simulink model "asg1_3k03"  (R2019a)
settings: Solver=FixedStepAuto  StartTime=0.0  StopTime=100  FixedStep=1e-3  RelTol=1e-3  EnableMultiTasking=on
undefined symbols (not defined in the file): D0, D1, D10, D11, D12, D13, D2, D3, D4, D5, D6, D7, D8, D9, PTA0, PTA1, PTA2, PTB23, PTB9, PTC16, PTC17, PTC2, PTC3, PTC4, PTD0, PTD1, PTD2, PTD3, sigbuilder_block
libraries: frdmk64flib x20
settings Model: SimulationMode=external  ExtModeTrigDuration=5  Creator=Jinge Li  LastModifiedBy=Junbo Huang
settings DataIOCC: ReturnWorkspaceOutputs=off
settings OptimizationCC: EnhancedBackFolding=on  PassReuseOutputArgsAs=Individual arguments  MaxStackSize=64  OptimizeBlockOrder=speed  DifferentSizesBufferReuse=on  OptimizationCustomize=off
settings DebuggingCC: ParameterTunabilityLossMsg=error  ArithmeticOperatorsInVariantConditions=warning
settings HardwareCC: ProdBitPerPointer=32  ProdBitPerSizeT=32  ProdBitPerPtrDiffT=32  ProdLargestAtomicInteger=Long  ProdLargestAtomicFloat=Double  ProdWordSize=32  ProdHWDeviceType=ARM Compatible->ARM Cortex
settings SFSimCC: MATLABDynamicMemAlloc=off
settings RTWCC: SystemTargetFile=ert.tlc  HardwareBoard=NXP FRDM-K64F  TLCOptions="-aInlineSetEventsForThisBaseRateFcn=TLC_FALSE -aSuppressMultiTaskScheduler=TLC_FALSE  -aRateBasedStepFcn=0"  TemplateMakefile=ert_default_tmf  GenerateReport=on  Toolchain=GNU Tools for ARM Embedded Processors  IncludeHyperlinkInReport=on  LaunchReport=on  GenerateTraceInfo=on  GenerateTraceReport=on  GenerateTraceReportSl=on  GenerateTraceReportSf=on  GenerateTraceReportEml=on
settings CodeAppCC: ForceParamTrailComments=on  IgnoreCustomStorageClasses=off  OperatorAnnotations=on  SimulinkDataObjDesc=on  SFDataObjDesc=on  InsertBlockDesc=on
settings ERTTargetCC: SupportContinuousTime=on  ExtMode=on  ExtModeTransport=4  ExtModeMexFile=sendToCommService  ExtModeMexArgs='asg1_3k03' 0

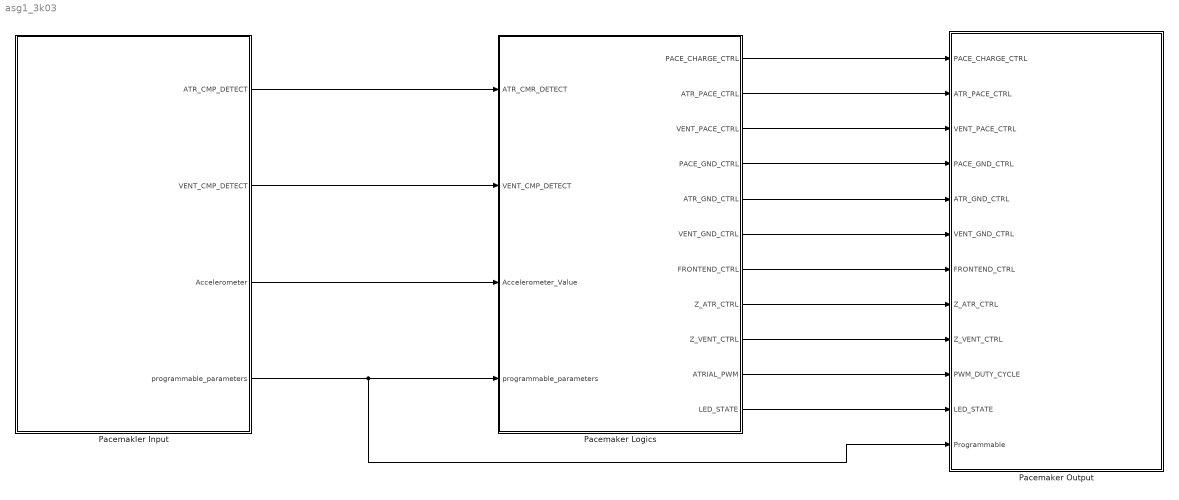
== system asg1_3k03 ==
  Pacemaker Logics : Subsystem
  Pacemaker Output : Subsystem
  Pacemakler Input : Subsystem
  wires:
  Pacemaker Logics/1(PACE_CHARGE_CTRL) -> Pacemaker Output/1(PACE_CHARGE_CTRL)
  Pacemaker Logics/3(VENT_PACE_CTRL) -> Pacemaker Output/3(VENT_PACE_CTRL)
  Pacemaker Logics/4(PACE_GND_CTRL) -> Pacemaker Output/4(PACE_GND_CTRL)
  Pacemaker Logics/5(ATR_GND_CTRL) -> Pacemaker Output/5(ATR_GND_CTRL)
  Pacemaker Logics/6(VENT_GND_CTRL) -> Pacemaker Output/6(VENT_GND_CTRL)
  Pacemakler Input/1(ATR_CMP_DETECT) -> Pacemaker Logics/1(ATR_CMR_DETECT)
  Pacemakler Input/2(VENT_CMP_DETECT) -> Pacemaker Logics/2(VENT_CMP_DETECT)
  Pacemaker Logics/2(ATR_PACE_CTRL) -> Pacemaker Output/2(ATR_PACE_CTRL)
  Pacemaker Logics/7(FRONTEND_CTRL) -> Pacemaker Output/7(FRONTEND_CTRL)
  Pacemakler Input/4(programmable_parameters) -> Pacemaker Output/12("Programmable "), Pacemaker Logics/4(programmable_parameters)
  Pacemaker Logics/8(Z_ATR_CTRL) -> Pacemaker Output/8(Z_ATR_CTRL)
  Pacemaker Logics/9(Z_VENT_CTRL) -> Pacemaker Output/9(Z_VENT_CTRL)
  Pacemaker Logics/10(ATRIAL_PWM) -> Pacemaker Output/10(PWM_DUTY_CYCLE)
  Pacemakler Input/3("Accelerometer ") -> Pacemaker Logics/3(Accelerometer_Value)
  Pacemaker Logics/11(LED_STATE) -> Pacemaker Output/11(LED_STATE)

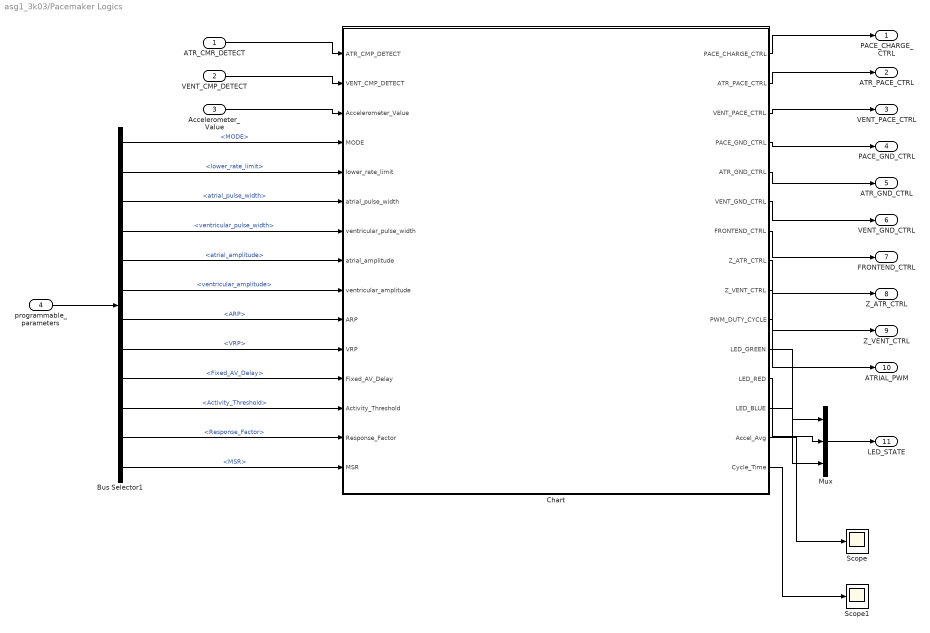
== system asg1_3k03/Pacemaker Logics ==
  ATR_CMR_DETECT : Inport
  VENT_CMP_DETECT : Inport  Port=2
  Accelerometer_Value : Inport  Port=3
  programmable_parameters : Inport  Port=4
  Bus Selector1 : BusSelector  OutputSignals=MODE,lower_rate_limit,atrial_pulse_width,ventricular_pulse_width,atrial_amplitude,ventricular_amplitude,ARP,VRP,Fixed_AV_Delay,Activity_Threshold,Response_Factor,MSR
  Chart : Stateflow chart  TreatAsAtomicUnit=on
  Mux : Mux  Inputs=3
  Scope : Scope
  Scope1 : Scope
  PACE_CHARGE_CTRL : Outport
  ATR_PACE_CTRL : Outport  Port=2
  VENT_PACE_CTRL : Outport  Port=3
  PACE_GND_CTRL : Outport  Port=4
  ATR_GND_CTRL : Outport  Port=5
  VENT_GND_CTRL : Outport  Port=6
  FRONTEND_CTRL : Outport  Port=7
  Z_ATR_CTRL : Outport  Port=8
  Z_VENT_CTRL : Outport  Port=9
  ATRIAL_PWM : Outport  Port=10
  LED_STATE : Outport  Port=11
  wires:
  Chart/1(PACE_CHARGE_CTRL) -> PACE_CHARGE_CTRL/1
  Bus Selector1/7 -> Chart/10(ARP)  "<ARP>"
  Bus Selector1/8 -> Chart/11(VRP)  "<VRP>"
  Bus Selector1/4 -> Chart/7(ventricular_pulse_width)  "<ventricular_pulse_width>"
  Chart/2(ATR_PACE_CTRL) -> ATR_PACE_CTRL/1
  Bus Selector1/6 -> Chart/9(ventricular_amplitude)  "<ventricular_amplitude>"
  Bus Selector1/5 -> Chart/8(atrial_amplitude)  "<atrial_amplitude>"
  Bus Selector1/2 -> Chart/5(lower_rate_limit)  "<lower_rate_limit>"
  Chart/9(Z_VENT_CTRL) -> Z_VENT_CTRL/1
  Chart/8(Z_ATR_CTRL) -> Z_ATR_CTRL/1
  Chart/7(FRONTEND_CTRL) -> FRONTEND_CTRL/1
  programmable_parameters/1 -> Bus Selector1/1
  Bus Selector1/1 -> Chart/4(MODE)  "<MODE>"
  Bus Selector1/3 -> Chart/6(atrial_pulse_width)  "<atrial_pulse_width>"
  VENT_CMP_DETECT/1 -> Chart/2(VENT_CMP_DETECT)
  Chart/4(PACE_GND_CTRL) -> PACE_GND_CTRL/1
  Chart/5(ATR_GND_CTRL) -> ATR_GND_CTRL/1
  Chart/6(VENT_GND_CTRL) -> VENT_GND_CTRL/1
  ATR_CMR_DETECT/1 -> Chart/1(ATR_CMP_DETECT)
  Chart/3(VENT_PACE_CTRL) -> VENT_PACE_CTRL/1
  Chart/10(PWM_DUTY_CYCLE) -> ATRIAL_PWM/1
  Bus Selector1/9 -> Chart/12(Fixed_AV_Delay)  "<Fixed_AV_Delay>"
  Accelerometer_Value/1 -> Chart/3(Accelerometer_Value)
  Chart/11(LED_GREEN) -> Mux/1
  Chart/12(LED_RED) -> Mux/2
  Chart/13(LED_BLUE) -> Mux/3
  Mux/1 -> LED_STATE/1
  Bus Selector1/10 -> Chart/13(Activity_Threshold)  "<Activity_Threshold>"
  Bus Selector1/11 -> Chart/14(Response_Factor)  "<Response_Factor>"
  Chart/14(Accel_Avg) -> Scope/1
  Bus Selector1/12 -> Chart/15(MSR)  "<MSR>"
  Chart/15(Cycle_Time) -> Scope1/1

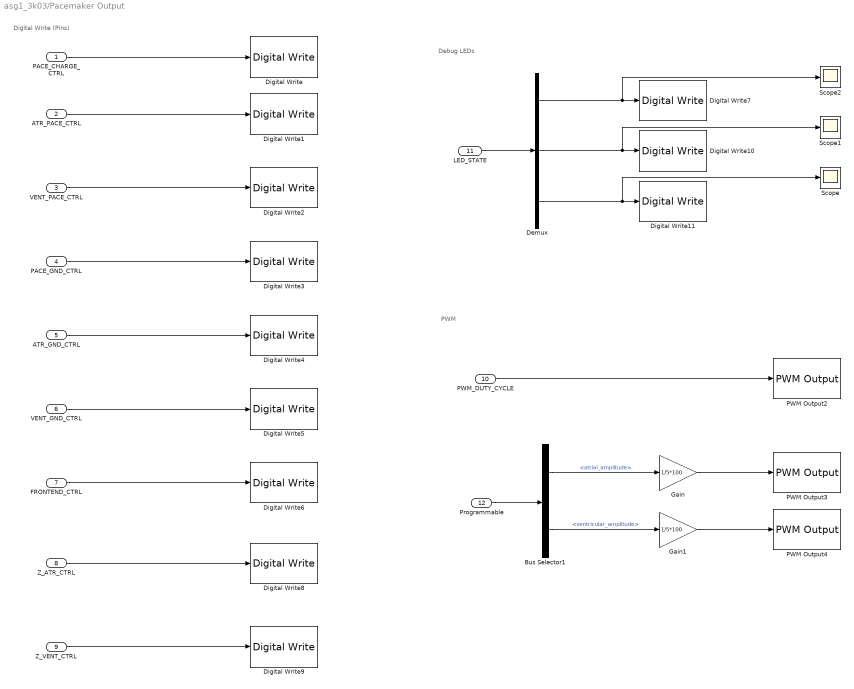
== system asg1_3k03/Pacemaker Output ==
  note: Digital Write (Pins)
  note: PWM
  note: Debug LEDs
  PACE_CHARGE_CTRL : Inport
  ATR_PACE_CTRL : Inport  Port=2
  VENT_PACE_CTRL : Inport  Port=3
  PACE_GND_CTRL : Inport  Port=4
  ATR_GND_CTRL : Inport  Port=5
  VENT_GND_CTRL : Inport  Port=6
  FRONTEND_CTRL : Inport  Port=7
  Z_ATR_CTRL : Inport  Port=8
  Z_VENT_CTRL : Inport  Port=9
  PWM_DUTY_CYCLE : Inport  Port=10
  LED_STATE : Inport  Port=11
  "Programmable " : Inport  Port=12
  Bus Selector1 : BusSelector  OutputSignals=atrial_amplitude,ventricular_amplitude
  Demux : Demux  Outputs=3
  Digital Write : frdmk64flib/Digital Write  Whichpin=PTB9 (D2)
      settings: SourceProductName=Simulink Coder Support Package for NXP FRDM-K64F Board
  Digital Write1 : frdmk64flib/Digital Write  Whichpin=PTA0 (D8)
      settings: SourceProductName=Simulink Coder Support Package for NXP FRDM-K64F Board
  Digital Write10 : frdmk64flib/Digital Write  Whichpin=RED_LED
      settings: SourceProductName=Simulink Coder Support Package for NXP FRDM-K64F Board
  Digital Write11 : frdmk64flib/Digital Write  Whichpin=BLUE_LED
      settings: SourceProductName=Simulink Coder Support Package for NXP FRDM-K64F Board
  Digital Write2 : frdmk64flib/Digital Write  Whichpin=PTC4 (D9)
      settings: SourceProductName=Simulink Coder Support Package for NXP FRDM-K64F Board
  Digital Write3 : frdmk64flib/Digital Write  Whichpin=PTD0 (D10)
      settings: SourceProductName=Simulink Coder Support Package for NXP FRDM-K64F Board
  Digital Write4 : frdmk64flib/Digital Write  Whichpin=PTD2 (D11)
      settings: SourceProductName=Simulink Coder Support Package for NXP FRDM-K64F Board
  Digital Write5 : frdmk64flib/Digital Write  Whichpin=PTD3 (D12)
      settings: SourceProductName=Simulink Coder Support Package for NXP FRDM-K64F Board
  Digital Write6 : frdmk64flib/Digital Write  Whichpin=PTD1 (D13)
      settings: SourceProductName=Simulink Coder Support Package for NXP FRDM-K64F Board
  Digital Write7 : frdmk64flib/Digital Write  Whichpin=GREEN_LED
      settings: SourceProductName=Simulink Coder Support Package for NXP FRDM-K64F Board
  Digital Write8 : frdmk64flib/Digital Write  Whichpin=PTB23 (D4)
      settings: SourceProductName=Simulink Coder Support Package for NXP FRDM-K64F Board
  Digital Write9 : frdmk64flib/Digital Write  Whichpin=PTC3 (D7)
      settings: SourceProductName=Simulink Coder Support Package for NXP FRDM-K64F Board
  Gain : Gain  Gain=1/5*100
  Gain1 : Gain  Gain=1/5*100
  PWM Output2 : frdmk64flib/PWM Output  Whichpin=PTA2 (D5)  InitialFrequency=2000  InitialDutyCycle=0
      settings: SourceProductName=Simulink Coder Support Package for NXP FRDM-K64F Board
  PWM Output3 : frdmk64flib/PWM Output  Whichpin=PTC2 (D6)  InitialFrequency=2000  InitialDutyCycle=0
      settings: SourceProductName=Simulink Coder Support Package for NXP FRDM-K64F Board
  PWM Output4 : frdmk64flib/PWM Output  Whichpin=PTA1 (D3)  InitialFrequency=2000  InitialDutyCycle=0
      settings: SourceProductName=Simulink Coder Support Package for NXP FRDM-K64F Board
  Scope : Scope
  Scope1 : Scope
  Scope2 : Scope
  wires:
  PACE_CHARGE_CTRL/1 -> Digital Write/1
  FRONTEND_CTRL/1 -> Digital Write6/1
  ATR_PACE_CTRL/1 -> Digital Write1/1
  VENT_PACE_CTRL/1 -> Digital Write2/1
  PACE_GND_CTRL/1 -> Digital Write3/1
  ATR_GND_CTRL/1 -> Digital Write4/1
  VENT_GND_CTRL/1 -> Digital Write5/1
  Z_ATR_CTRL/1 -> Digital Write8/1
  Z_VENT_CTRL/1 -> Digital Write9/1
  Bus Selector1/1 -> Gain/1  "<atrial_amplitude>"
  Bus Selector1/2 -> Gain1/1  "<ventricular_amplitude>"
  "Programmable "/1 -> Bus Selector1/1
  PWM_DUTY_CYCLE/1 -> PWM Output2/1
  Gain/1 -> PWM Output3/1
  Gain1/1 -> PWM Output4/1
  Demux/3 -> Scope/1, Digital Write11/1
  LED_STATE/1 -> Demux/1
  Demux/1 -> Scope2/1, Digital Write7/1
  Demux/2 -> Scope1/1, Digital Write10/1

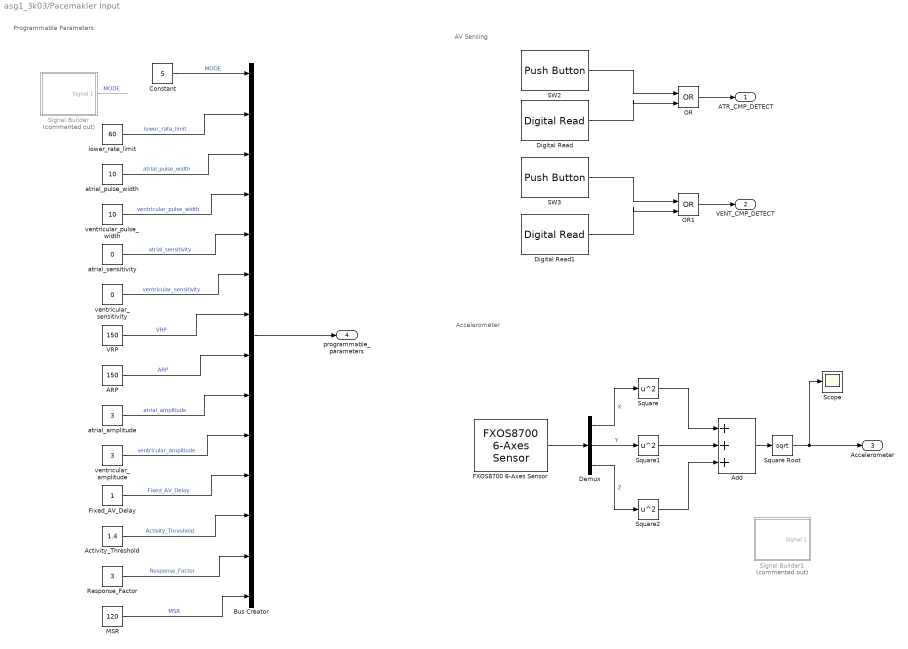
== system asg1_3k03/Pacemakler Input ==
  note: Accelerometer
  note: Programmable Parameters
  note: AV Sensing
  ARP : Constant  Value=150
  Activity_Threshold : Constant  Value=1.4
  Add : Sum  Inputs=+++
  Bus Creator : BusCreator  Inputs=14
  Constant : Constant  Value=5
  Demux : Demux  Outputs=3
  Digital Read : frdmk64flib/Digital Read  Whichpin=PTC16 (D0)  SampleTime=-1
      settings: SourceProductName=Simulink Coder Support Package for NXP FRDM-K64F Board
  Digital Read1 : frdmk64flib/Digital Read  Whichpin=PTC17 (D1)  SampleTime=-1
      settings: SourceProductName=Simulink Coder Support Package for NXP FRDM-K64F Board
  FXOS8700 6-Axes Sensor : frdmk64flib/FXOS8700 6-Axes Sensor  Activesensor=Accelerometer only  ODR=800Hz  HybridODR=400Hz  Accelfullrange=-4g to +4g  SampleTime=-1
      settings: SourceProductName=Simulink Coder Support Package for NXP FRDM-K64F Board
  Fixed_AV_Delay : Constant
  "MSR " : Constant  Value=120
  OR : Logic  Operator=OR  IconShape=distinctive  AllPortsSameDT=off  OutDataTypeStr=boolean
  OR1 : Logic  Operator=OR  IconShape=distinctive  AllPortsSameDT=off  OutDataTypeStr=boolean
  Response_Factor : Constant  Value=3
  SW2 : frdmk64flib/Push Button  Whichswitch=SW2  SampleTime1=-1
      settings: SourceProductName=Simulink Coder Support Package for NXP FRDM-K64F Board
  SW3 : frdmk64flib/Push Button  Whichswitch=SW3  SampleTime1=-1
      settings: SourceProductName=Simulink Coder Support Package for NXP FRDM-K64F Board
  Scope : Scope
  Signal Builder : Subsystem  Tag=STV Subsys  Commented=on  LoadFcn=sigbuilder_block('load');  StartFcn=sigbuilder_block('start');  StopFcn=sigbuilder_block('stop');  ClipboardFcn=sigbuilder_block('clipboard');  mask(Sigbuilder block){tuvar=[0:10]}
      mask help: Simulink:masks:SigbuilderBlock_MD
      mask init:
      | if ~strcmp(get_param(bdroot(gcbh),'SimulationStatus'),'stopped') tuvar = sigbuilder_block('maskInit'); end
      settings: CopyFcn=sigbuilder_block('copy');  DeleteFcn=sigbuilder_block('delete');  ModelCloseFcn=sigbuilder_block('modelClose');  PreSaveFcn=sigbuilder_block('preSave');  PauseFcn=sigbuilder_block('pause');  ContinueFcn=sigbuilder_block('continue');  NameChangeFcn=sigbuilder_block('namechange');  OpenFcn=sigbuilder_block('open',[347.5 209 550.5 400 ]);  CloseFcn=sigbuilder_block('close');
      mask Display: plot(0, 0, 100, 100,[2, 2, 32, 32, 2], [68, 8, 8, 68, 68],[32, 2], [38, 38], [32, 19, 2],[53, 60, 44], [32, 17, 17, 2],[16, 16, 31, 31]);txt = getActiveGroup(gcbh);text(2, 100, txt,'verticalAlignment', 'top');
  Signal Builder1 : Subsystem  Tag=STV Subsys  Commented=on  LoadFcn=sigbuilder_block('load');  StartFcn=sigbuilder_block('start');  StopFcn=sigbuilder_block('stop');  ClipboardFcn=sigbuilder_block('clipboard');  mask(Sigbuilder block){tuvar=[0:10]}
      mask help: Simulink:masks:SigbuilderBlock_MD
      mask init:
      | if ~strcmp(get_param(bdroot(gcbh),'SimulationStatus'),'stopped') tuvar = sigbuilder_block('maskInit'); end
      settings: CopyFcn=sigbuilder_block('copy');  DeleteFcn=sigbuilder_block('delete');  ModelCloseFcn=sigbuilder_block('modelClose');  PreSaveFcn=sigbuilder_block('preSave');  PauseFcn=sigbuilder_block('pause');  ContinueFcn=sigbuilder_block('continue');  NameChangeFcn=sigbuilder_block('namechange');  OpenFcn=sigbuilder_block('open',[347.5 209 550.5 400 ]);  CloseFcn=sigbuilder_block('close');
      mask Display: plot(0, 0, 100, 100,[2, 2, 32, 32, 2], [68, 8, 8, 68, 68],[32, 2], [38, 38], [32, 19, 2],[53, 60, 44], [32, 17, 17, 2],[16, 16, 31, 31]);txt = getActiveGroup(gcbh);text(2, 100, txt,'verticalAlignment', 'top');
  Square : Math  Operator=square  SaturateOnIntegerOverflow=on
  Square Root : Sqrt  SaturateOnIntegerOverflow=on
  Square1 : Math  Operator=square  SaturateOnIntegerOverflow=on
  Square2 : Math  Operator=square  SaturateOnIntegerOverflow=on
  VRP : Constant  Value=150
  atrial_amplitude : Constant  Value=3
  atrial_pulse_width : Constant  Value=10
  atrial_sensitivity : Constant  Value=0
  lower_rate_limit : Constant  Value=60
  ventricular_amplitude : Constant  Value=3
  ventricular_pulse_width : Constant  Value=10
  ventricular_sensitivity : Constant  Value=0
  ATR_CMP_DETECT : Outport
  VENT_CMP_DETECT : Outport  Port=2
  "Accelerometer " : Outport  Port=3
  programmable_parameters : Outport  Port=4
  wires:
  OR/1 -> ATR_CMP_DETECT/1
  SW2/1 -> OR/1
  Digital Read/1 -> OR/2
  OR1/1 -> VENT_CMP_DETECT/1
  SW3/1 -> OR1/1
  Digital Read1/1 -> OR1/2
  Signal Builder/1(Signal 1) -> ?  "MODE"
  Bus Creator/1 -> programmable_parameters/1
  lower_rate_limit/1 -> Bus Creator/2  "lower_rate_limit"
  atrial_pulse_width/1 -> Bus Creator/3  "atrial_pulse_width"
  ventricular_pulse_width/1 -> Bus Creator/4  "ventricular_pulse_width"
  atrial_sensitivity/1 -> Bus Creator/5  "atrial_sensitivity"
  ventricular_sensitivity/1 -> Bus Creator/6  "ventricular_sensitivity"
  VRP/1 -> Bus Creator/7  "VRP"
  ARP/1 -> Bus Creator/8  "ARP"
  atrial_amplitude/1 -> Bus Creator/9  "atrial_amplitude"
  ventricular_amplitude/1 -> Bus Creator/10  "ventricular_amplitude"
  Fixed_AV_Delay/1 -> Bus Creator/11  "Fixed_AV_Delay"
  FXOS8700 6-Axes Sensor/1 -> Demux/1
  Demux/1 -> Square/1  "X"
  Demux/2 -> Square1/1  "Y"
  Demux/3 -> Square2/1  "Z"
  Square/1 -> Add/1
  Square1/1 -> Add/2
  Square2/1 -> Add/3
  Add/1 -> Square Root/1
  Square Root/1 -> Scope/1, "Accelerometer "/1
  Constant/1 -> Bus Creator/1  "MODE"
  Activity_Threshold/1 -> Bus Creator/12  "Activity_Threshold"
  Response_Factor/1 -> Bus Creator/13  "Response_Factor"
  "MSR "/1 -> Bus Creator/14  "MSR"

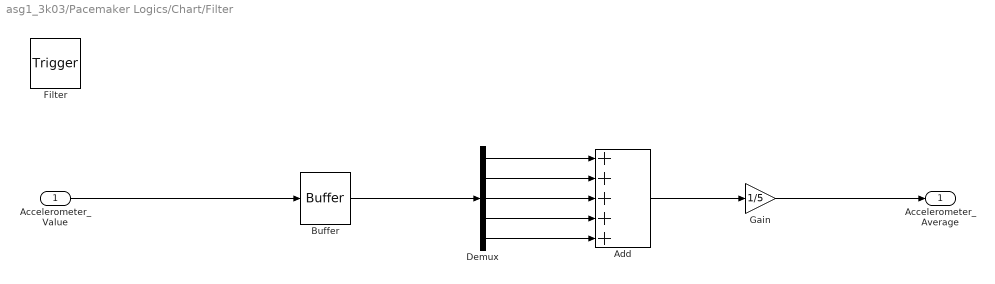
== system asg1_3k03/Pacemaker Logics/Chart/Filter ==
  Accelerometer_Value : Inport  OutDataTypeStr=double  PortDimensions=1
  "Filter " : TriggerPort  TriggerType=function-call  VariantControl=(inherit)
      settings: CopyFcn=Stateflow.SLINSF.SimulinkMan.removeBlockPreDeleteFcn  PreDeleteFcn=Stateflow.SLINSF.SimulinkMan.unsafePredeleteFcn
  Add : Sum  Inputs=+++++
  Buffer : Buffer  N=5  V=4  ic=1  OutputFrames=off
  Demux : Demux  Outputs=5
  Gain : Gain  Gain=1/5
  Accelerometer_Average : Outport
  wires:
  Accelerometer_Value/1 -> Buffer/1
  Buffer/1 -> Demux/1
  Demux/1 -> Add/1
  Demux/2 -> Add/2
  Demux/3 -> Add/3
  Demux/4 -> Add/4
  Demux/5 -> Add/5
  Add/1 -> Gain/1
  Gain/1 -> Accelerometer_Average/1

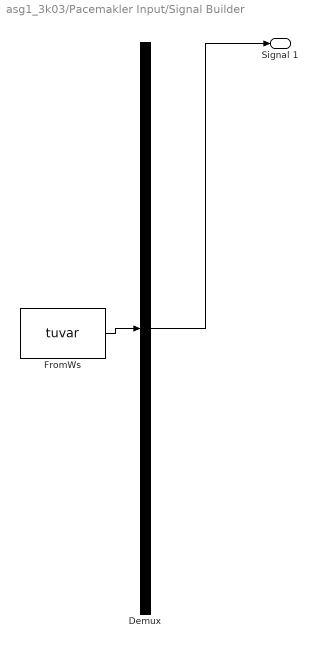
== system asg1_3k03/Pacemakler Input/Signal Builder ==
  Demux : Demux  Tag=STV Demux  Outputs=1
  FromWs : FromWorkspace  Tag=STV FromWs  VariableName=tuvar  SampleTime=0
      SigBuilderData=|
      | common.afterFinalStr = 'Extrapolate'
      | common.sampleTime = 0
      | dataSet.timeRange = [0 60]
      | dataSet.name = 'Group 1'
      | sbobj.Groups.Name = 'Group 1'
      | sbobj.Groups.Signals.Name = 'Signal 1'
      | sbobj.Groups.Signals.XData = [0 4.6 4.6 10.9 10.9 60]
      | sbobj.Groups.Signals.YData = [4 4 3 3 2 2]
      | sbobj.Groups.TimeRange = [0 60]
  Signal 1 : Outport  Tag=STV Outport
  wires:
  Demux/1 -> Signal 1/1
  FromWs/1 -> Demux/1

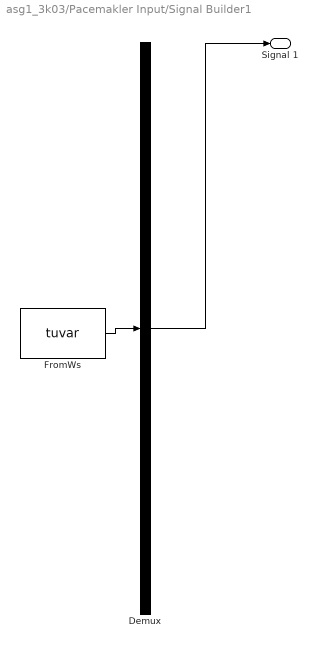
== system asg1_3k03/Pacemakler Input/Signal Builder1 ==
  Demux : Demux  Tag=STV Demux  Outputs=1
  FromWs : FromWorkspace  Tag=STV FromWs  VariableName=tuvar  SampleTime=0
      SigBuilderData=|
      | common.afterFinalStr = 'Extrapolate'
      | common.sampleTime = 0
      | dataSet.timeRange = [0 60]
      | dataSet.name = 'Group 1'
      | sbobj.Groups.Name = 'Group 1'
      | sbobj.Groups.Signals.Name = 'Signal 1'
      | sbobj.Groups.Signals.XData = [0 4.6 4.6 10.9 10.9 60]
      | sbobj.Groups.Signals.YData = [2.51 2.51 3.5 3.5 1.85 1.85]
      | sbobj.Groups.TimeRange = [0 60]
  Signal 1 : Outport  Tag=STV Outport
  wires:
  Demux/1 -> Signal 1/1
  FromWs/1 -> Demux/1

== stateflow chart asg1_3k03/Pacemaker Logics/Chart ==
  state VOO_MODE
    note: Charge up C22 and discharge C21 to ground
    note: Discharge C22 to C21 which charge up C21
    state VOO_CHARGE
      entry:
      PACE_CHARGE_CTRL = true;
      VENT_PACE_CTRL = false;
      VENT_GND_CTRL = true;
      PACE_GND_CTRL = true;
      Z_ATR_CTRL = false;
      Z_VENT_CTRL = false;
      %Cycle_Time = Cycle_Min;
    state VOO_PACE
      entry:
      PACE_CHARGE_CTRL = false;
      VENT_PACE_CTRL = true;
      VENT_GND_CTRL = false;
      PACE_GND_CTRL = true;
      Z_ATR_CTRL = false;
      Z_VENT_CTRL = false;
      PWM_DUTY_CYCLE = (ventricular_amplitude/5)*100;
    VOO_MODE.VOO_CHARGE -> VOO_MODE.VOO_PACE : after((60/lower_rate_limit)*1000 - ventricular_pulse_width,msec)
    VOO_MODE.VOO_PACE -> VOO_MODE.VOO_CHARGE : after(ventricular_pulse_width,msec)
  state VOOR_MODE
    note: Charge up C22 and discharge C21 to ground
    note: Discharge C22 to C21 which charge up C21
    state VOO_PACE
      entry:
      PACE_CHARGE_CTRL = false;
      VENT_PACE_CTRL = true;
      VENT_GND_CTRL = false;
      PACE_GND_CTRL = true;
      Z_ATR_CTRL = false;
      Z_VENT_CTRL = false;
      PWM_DUTY_CYCLE = (ventricular_amplitude/5)*100;
      LED_GREEN = 1;
    state VOO_CHARGE
      entry:
      PACE_CHARGE_CTRL = true;
      VENT_PACE_CTRL = false;
      VENT_GND_CTRL = true;
      PACE_GND_CTRL = true;
      Z_ATR_CTRL = false;
      Z_VENT_CTRL = false;
    state Filter
      entry:
      LED_GREEN = 0;
      Accel_Avg = Filter(Accelerometer_Value);
    state Rate_Adaptive
      entry:
      Cycle_Time = rateConversion(Cycle_Min, Cycle_Max, Response_Factor, Activity_Threshold, Accelerometer_Value);
    VOOR_MODE.VOO_CHARGE -> VOOR_MODE.VOO_PACE : after(Cycle_Time - ventricular_pulse_width,msec)
    VOOR_MODE.VOO_PACE -> Filter : after(ventricular_pulse_width,msec)
    Rate_Adaptive -> VOOR_MODE.VOO_CHARGE
    Filter -> Rate_Adaptive
  state Accelerometer_Average = Filter(Accelerometer_Value) [function]
  note: Starting state, open all the switchs for safety
  note: VOO Mode
  state AOO_MODE
    note: Charge up C22 and discharge C21 to ground
    note: Discharge C22 to C21 which charge up C21
    state AOO_CHARGE
      entry:
      PACE_CHARGE_CTRL = true;
      %charge C22
      ATR_PACE_CTRL = false;
      ATR_GND_CTRL = true;
      PACE_GND_CTRL = true;
      %discharge C21
      Z_ATR_CTRL = false;
      Z_VENT_CTRL = false;
    state AOO_PACE
      entry:
      PACE_CHARGE_CTRL = false;
      PACE_GND_CTRL = true; %charge C21
      ATR_PACE_CTRL = true; %discharge C22
      ATR_GND_CTRL = false;
      Z_ATR_CTRL = false;
      Z_VENT_CTRL = false;
      PWM_DUTY_CYCLE = (atrial_amplitude/5)*100;
      %set PWM duty cycle based on input amplitude
    note: Lower rate limit is converted to period of cycle
    note: Pace for the period specified by pulse width
    AOO_MODE.AOO_CHARGE -> AOO_MODE.AOO_PACE : after((60/lower_rate_limit)*1000 - atrial_pulse_width,msec)
    AOO_MODE.AOO_PACE -> AOO_MODE.AOO_CHARGE : after(atrial_pulse_width,msec)
  state AOOR_MODE
    note: Charge up C22 and discharge C21 to ground
    note: Discharge C22 to C21 which charge up C21
    state AOO_CHARGE
      entry:
      PACE_CHARGE_CTRL = true;
      %charge C22
      ATR_PACE_CTRL = false;
      ATR_GND_CTRL = true;
      PACE_GND_CTRL = true;
      %discharge C21
      Z_ATR_CTRL = false;
      Z_VENT_CTRL = false;
    state AOO_PACE
      entry:
      PACE_CHARGE_CTRL = false;
      PACE_GND_CTRL = true; %charge C21
      ATR_PACE_CTRL = true; %discharge C22
      ATR_GND_CTRL = false;
      Z_ATR_CTRL = false;
      Z_VENT_CTRL = false;
      PWM_DUTY_CYCLE = (atrial_amplitude/5)*100;
      %set PWM duty cycle based on input amplitude
    note: Lower rate limit is converted to period of cycle
    note: Pace for the period specified by pulse width
    AOOR_MODE.AOO_CHARGE -> AOOR_MODE.AOO_PACE : after((60/lower_rate_limit)*1000 - atrial_pulse_width,msec)
    AOOR_MODE.AOO_PACE -> AOOR_MODE.AOO_CHARGE : after(atrial_pulse_width,msec)
  state MAIN
    entry:
    PACE_CHARGE_CTRL = false;
    VENT_PACE_CTRL = false;
    ATR_PACE_CTRL = false;
    VENT_GND_CTRL = false;
    ATR_GND_CTRL = false;
    PACE_GND_CTRL = false;
    FRONTEND_CTRL = false;
    Z_ATR_CTRL = false;
    Z_VENT_CTRL = false;
    Cycle_Max = (60/lower_rate_limit)*1000;
    Cycle_Min = (60/MSR)*1000;
    Cycle_Time = Cycle_Max;
    %%
    LED_GREEN = 0;
    LED_RED = 0;
    LED_BLUE = 0;
  note: AOO Mode
  note: MODE
      | Mode Name
      |
      | 0
      | VOO
      |
      | 1
      | AOO
      |
      | 2
      | VVI
      |
      | 3
      | AAI
      |
      | 4
      | DOO
      |
      | 5
      | VOOR
      |
      | 6
      | AOOR
      |
      | 7
      | VVIR
      |
      | 8
      | AAIR
      |
      | 9
      | DOOR
  state VVI_MODE
    note: Charge up C22 and discharge C21 to ground, sensing natrual signal
    note: Discharge C22 to C21 which charge up C21
    state VVI_CHARGE
      entry:
      FRONTEND_CTRL = true;
      PACE_CHARGE_CTRL = true;
      VENT_PACE_CTRL = false;
      VENT_GND_CTRL = true;
      PACE_GND_CTRL = true;
      Z_ATR_CTRL = false;
      Z_VENT_CTRL = false;
    state VVI_PACE
      entry:
      PACE_CHARGE_CTRL = false;
      VENT_PACE_CTRL = true;
      VENT_GND_CTRL = false;
      PACE_GND_CTRL = true;
      Z_ATR_CTRL = false;
      Z_VENT_CTRL = false;
      PWM_DUTY_CYCLE =  (ventricular_amplitude/5)*100;
      LED_GREEN = 1;
    note: Signal detected, refresh VRP counting
    note: Refractory Period
    state VVI_DETECTED
      FRONTEND_CTRL = false;
      %stay in this state during the ...
      %refractory period
      PACE_CHARGE_CTRL = true;
      VENT_PACE_CTRL = false;
      VENT_GND_CTRL = true;
      PACE_GND_CTRL = true;
      Z_ATR_CTRL = false;
      Z_VENT_CTRL = false;
      LED_GREEN = 0;
    note: Inhibit
    VVI_MODE.VVI_CHARGE -> VVI_MODE.VVI_PACE [order 2] : after((60/lower_rate_limit)*1000 - VRP - ventricular_pulse_width,msec)
    VVI_MODE.VVI_PACE -> VVI_MODE.VVI_DETECTED : after(ventricular_pulse_width,msec)
    VVI_MODE.VVI_CHARGE -> (junction 125) [order 1] : [VENT_CMP_DETECT == true]
    VVI_MODE.VVI_DETECTED -> VVI_MODE.VVI_CHARGE : after(VRP, msec)
    (junction 125) -> VVI_MODE.VVI_DETECTED : after(ventricular_pulse_width, msec)
  state VVIR_MODE
    note: Charge up C22 and discharge C21 to ground, sensing natrual signal
    note: Discharge C22 to C21 which charge up C21
    state VVI_CHARGE
      entry:
      FRONTEND_CTRL = true;
      PACE_CHARGE_CTRL = true;
      VENT_PACE_CTRL = false;
      VENT_GND_CTRL = true;
      PACE_GND_CTRL = true;
      Z_ATR_CTRL = false;
      Z_VENT_CTRL = false;
    state VVI_PACE
      entry:
      PACE_CHARGE_CTRL = false;
      VENT_PACE_CTRL = true;
      VENT_GND_CTRL = false;
      PACE_GND_CTRL = true;
      Z_ATR_CTRL = false;
      Z_VENT_CTRL = false;
      PWM_DUTY_CYCLE =  (ventricular_amplitude/5)*100;
    note: Signal detected, refresh VRP counting
    note: Refractory Period
    state VVI_DETECTED
      FRONTEND_CTRL = false;
      %stay in this state during the ...
      %refractory period
      PACE_CHARGE_CTRL = true;
      VENT_PACE_CTRL = false;
      VENT_GND_CTRL = true;
      PACE_GND_CTRL = true;
      Z_ATR_CTRL = false;
      Z_VENT_CTRL = false;
    note: Inhibit
    VVIR_MODE.VVI_CHARGE -> VVIR_MODE.VVI_PACE [order 2] : after((60/lower_rate_limit)*1000 - VRP - ventricular_pulse_width,msec)
    VVIR_MODE.VVI_PACE -> VVIR_MODE.VVI_DETECTED : after(ventricular_pulse_width,msec)
    VVIR_MODE.VVI_DETECTED -> VVIR_MODE.VVI_CHARGE : after(VRP, msec)
    VVIR_MODE.VVI_CHARGE -> (junction 271) [order 1] : [VENT_CMP_DETECT == true]
    (junction 271) -> VVIR_MODE.VVI_DETECTED : after(ventricular_pulse_width, msec)
  note: VVI Mode
  note: AAI Mode
  state AAIR_MODE
    note: Charge up C22 and discharge C21 to ground, sensing natrual signal
    note: Discharge C22 to C21 which charge up C21
    state AAI_CHARGE
      entry:
      FRONTEND_CTRL = true;
      PACE_CHARGE_CTRL = true;
      ATR_PACE_CTRL = false;
      ATR_GND_CTRL = true;
      PACE_GND_CTRL = true;
      Z_ATR_CTRL = false;
      Z_VENT_CTRL = false;
    state AAI_PACE
      entry:
      PACE_CHARGE_CTRL = false;
      ATR_PACE_CTRL = true;
      ATR_GND_CTRL = false;
      PACE_GND_CTRL = true;
      Z_ATR_CTRL = false;
      Z_VENT_CTRL = false;
      PWM_DUTY_CYCLE = (atrial_amplitude/5)*100;
    note: Signal detected, refresh ARP counting
    state AAI_DETECTED
      FRONTEND_CTRL = false;
      %stay in this state during the ...
      %refractory period
      PACE_CHARGE_CTRL = true;
      ATR_PACE_CTRL = false;
      ATR_GND_CTRL = true;
      PACE_GND_CTRL = true;
      Z_ATR_CTRL = false;
      Z_VENT_CTRL = false;
    note: Inhibit
    note: Refractory Period
    AAIR_MODE.AAI_CHARGE -> AAIR_MODE.AAI_PACE [order 2] : after((60/lower_rate_limit)*1000 - ARP - atrial_pulse_width,msec)
    AAIR_MODE.AAI_PACE -> AAIR_MODE.AAI_DETECTED : after(atrial_pulse_width,msec)
    AAIR_MODE.AAI_DETECTED -> AAIR_MODE.AAI_CHARGE : after(ARP,msec)
    AAIR_MODE.AAI_CHARGE -> (junction 245) [order 1] : [ATR_CMP_DETECT == true]
    (junction 245) -> AAIR_MODE.AAI_DETECTED : after(atrial_pulse_width, msec)
  state AAI_MODE
    note: Charge up C22 and discharge C21 to ground, sensing natrual signal
    note: Discharge C22 to C21 which charge up C21
    state AAI_CHARGE
      entry:
      FRONTEND_CTRL = true;
      PACE_CHARGE_CTRL = true;
      ATR_PACE_CTRL = false;
      ATR_GND_CTRL = true;
      PACE_GND_CTRL = true;
      Z_ATR_CTRL = false;
      Z_VENT_CTRL = false;
    state AAI_PACE
      entry:
      PACE_CHARGE_CTRL = false;
      ATR_PACE_CTRL = true;
      ATR_GND_CTRL = false;
      PACE_GND_CTRL = true;
      Z_ATR_CTRL = false;
      Z_VENT_CTRL = false;
      PWM_DUTY_CYCLE = (atrial_amplitude/5)*100;
      LED_RED = 1;
    note: Signal detected, refresh ARP counting
    state AAI_DETECTED
      FRONTEND_CTRL = false;
      %stay in this state during the ...
      %refractory period
      PACE_CHARGE_CTRL = true;
      ATR_PACE_CTRL = false;
      ATR_GND_CTRL = true;
      PACE_GND_CTRL = true;
      Z_ATR_CTRL = false;
      Z_VENT_CTRL = false;
      LED_RED = 0;
    note: Inhibit
    note: Refractory Period
    AAI_MODE.AAI_CHARGE -> AAI_MODE.AAI_PACE [order 2] : after((60/lower_rate_limit)*1000 - ARP - atrial_pulse_width,msec)
    AAI_MODE.AAI_PACE -> AAI_MODE.AAI_DETECTED : after(atrial_pulse_width,msec)
    AAI_MODE.AAI_CHARGE -> (junction 139) [order 1] : [ATR_CMP_DETECT == true]
    AAI_MODE.AAI_DETECTED -> AAI_MODE.AAI_CHARGE : after(ARP,msec)
    (junction 139) -> AAI_MODE.AAI_DETECTED : after(atrial_pulse_width, msec)
  note: DOO Mode
  state DOOR_MODE
    note: Charge up C22 and discharge C21 to ground
    note: Discharge C22 to C21 which charge up C21
    state DOO_CHARGE
      entry:
      PACE_CHARGE_CTRL = true;
      PACE_GND_CTRL = true;
      %Turn off both
      ATR_PACE_CTRL = false;
      ATR_GND_CTRL = true;
      VENT_PACE_CTRL = false;
      VENT_GND_CTRL = true;
      %%%
      Z_ATR_CTRL = false;
      Z_VENT_CTRL = false;
    state ATRIAL_PACE
      entry:
      PACE_CHARGE_CTRL = false;
      PACE_GND_CTRL = true;
      %Pace Atrium
      ATR_PACE_CTRL = true;
      ATR_GND_CTRL = false;
      %%
      Z_ATR_CTRL = false;
      Z_VENT_CTRL = false;
      PWM_DUTY_CYCLE = (atrial_amplitude/5)*100;
    state MODE_CHECK
    state VENT_PACE
      entry:
      PACE_CHARGE_CTRL = false;
      PACE_GND_CTRL = true;
      %charge C21
      VENT_PACE_CTRL = true;
      VENT_GND_CTRL = false;
      Z_ATR_CTRL = false;
      Z_VENT_CTRL = false;
      PWM_DUTY_CYCLE = (ventricular_amplitude/5)*100;
    state AV_Delay
      entry:
      ATR_PACE_CTRL = false;
      ATR_GND_CTRL = false;
    DOOR_MODE.DOO_CHARGE -> DOOR_MODE.ATRIAL_PACE [order 1] : after(Cycle_Time - atrial_pulse_width - ventricular_pulse_width - Fixed_AV_Delay ,msec)
    DOOR_MODE.DOO_CHARGE -> DOOR_MODE.MODE_CHECK [order 2] : [MODE ~= 4]
    DOOR_MODE.ATRIAL_PACE -> DOOR_MODE.AV_Delay : after(atrial_pulse_width, msec)
    DOOR_MODE.VENT_PACE -> DOOR_MODE.DOO_CHARGE : after(ventricular_pulse_width, msec)
    DOOR_MODE.AV_Delay -> DOOR_MODE.VENT_PACE : after(Fixed_AV_Delay, msec)
  state DOO_MODE
    note: Charge up C22 and discharge C21 to ground
    note: Discharge C22 to C21 which charge up C21
    state DOO_CHARGE
      entry:
      PACE_CHARGE_CTRL = true;
      PACE_GND_CTRL = true;
      %Turn off both
      ATR_PACE_CTRL = false;
      ATR_GND_CTRL = true;
      VENT_PACE_CTRL = false;
      VENT_GND_CTRL = true;
      %%%
      Z_ATR_CTRL = false;
      Z_VENT_CTRL = false;
      LED_BLUE = 0;
    state ATRIAL_PACE
      entry:
      PACE_CHARGE_CTRL = false;
      PACE_GND_CTRL = true;
      %Pace Atrium
      ATR_PACE_CTRL = true;
      ATR_GND_CTRL = false;
      %%
      Z_ATR_CTRL = false;
      Z_VENT_CTRL = false;
      PWM_DUTY_CYCLE = (atrial_amplitude/5)*100;
      LED_BLUE = 1;
    state MODE_CHECK
    state VENT_PACE
      entry:
      PACE_CHARGE_CTRL = false;
      PACE_GND_CTRL = true;
      %charge C21
      VENT_PACE_CTRL = true;
      VENT_GND_CTRL = false;
      Z_ATR_CTRL = false;
      Z_VENT_CTRL = false;
      PWM_DUTY_CYCLE = (ventricular_amplitude/5)*100;
    state AV_Delay
      entry:
      ATR_PACE_CTRL = false;
      ATR_GND_CTRL = false;
    DOO_MODE.DOO_CHARGE -> DOO_MODE.ATRIAL_PACE [order 1] : after(Cycle_Time - atrial_pulse_width - ventricular_pulse_width - Fixed_AV_Delay ,msec)
    DOO_MODE.DOO_CHARGE -> DOO_MODE.MODE_CHECK [order 2] : [MODE ~= 4]
    DOO_MODE.ATRIAL_PACE -> DOO_MODE.AV_Delay : after(atrial_pulse_width, msec)
    DOO_MODE.VENT_PACE -> DOO_MODE.DOO_CHARGE : after(ventricular_pulse_width, msec)
    DOO_MODE.AV_Delay -> DOO_MODE.VENT_PACE : after(Fixed_AV_Delay, msec)
  AAI_MODE.AAI_CHARGE -> MAIN [order 3] : [MODE ~= 3]
  VVI_MODE.VVI_CHARGE -> MAIN [order 3] : [MODE ~= 2]
  MAIN -> VOOR_MODE.VOO_CHARGE [order 6] : [MODE == 5]
  MAIN -> DOOR_MODE.DOO_CHARGE [order 10] : [MODE == 9]
  MAIN -> AAIR_MODE.AAI_CHARGE [order 9] : [MODE == 8]
  MAIN -> VVIR_MODE.VVI_CHARGE [order 8] : [MODE == 7]
  MAIN -> VOO_MODE.VOO_CHARGE [order 1] : [MODE == 0]
  (default) -> MAIN
  DOOR_MODE.MODE_CHECK -> MAIN
  DOO_MODE.MODE_CHECK -> MAIN
  MAIN -> AOOR_MODE.AOO_CHARGE [order 7] : [MODE == 6]
  MAIN -> AOO_MODE.AOO_CHARGE [order 2] : [MODE == 1]
  MAIN -> VVI_MODE.VVI_CHARGE [order 3] : [MODE == 2]
  MAIN -> AAI_MODE.AAI_CHARGE [order 4] : [MODE == 3]
  MAIN -> DOO_MODE.DOO_CHARGE [order 5] : [MODE == 4]
  data: Accelerometer_Value function_input double size=1; Accelerometer_Average function_output; Cycle_Low function_input; Cycle_High function_input; RF function_input; Atv_Threshold function_input; Acc_Avg function_input; Cycle function_output; ATR_CMP_DETECT input boolean; VENT_CMP_DETECT input boolean; Accelerometer_Value input; PACE_CHARGE_CTRL output boolean; ATR_PACE_CTRL output boolean; VENT_PACE_CTRL output boolean; PACE_GND_CTRL output boolean; ATR_GND_CTRL output boolean; VENT_GND_CTRL output boolean; FRONTEND_CTRL output boolean; MODE input double; lower_rate_limit input; atrial_pulse_width input; ventricular_pulse_width input; atrial_amplitude input; ventricular_amplitude input; ARP input; VRP input; Z_ATR_CTRL output boolean; Z_VENT_CTRL output boolean; PWM_DUTY_CYCLE output double; Fixed_AV_Delay input; LED_GREEN output int16; LED_RED output int16; LED_BLUE output int16; Activity_Threshold input; Response_Factor input; Accel_Avg output double; MSR input; Cycle_Min local; Cycle_Max local; Cycle_Time output
  function Cycle = rateConversion(Cycle_Low, Cycle_High, RF, Atv_Threshold, Acc_Avg):
    | function Cycle = rateConversion(Cycle_Low, Cycle_High, RF, Atv_Threshold, Acc_Avg)
    |     
    |     if Acc_Avg <= Atv_Threshold
    |         Cycle = Cycle_High;
    |         return;
    |     end    
    |    
    |     Delta_Y = Cycle_High - Cycle_Low;
    |     RF_FACTOR = (RF - 1)/(16 - 1);
    |     Max_Activity_Offset = 4;
    |     Min_Activity_Offset = 1;
    |     Delta_X = Min_Activity_Offset + (Max_Activity_Offset - Min_Activity_Offset)*RF_FACTOR;
    |     Slope = Delta_Y/Delta_X;
    | 
    |     Cycle = Cycle_High -  Slope * (Acc_Avg - Atv_Threshold);
    |     
    |     if Cycle <= Cycle_Low
    |         Cycle = Cycle_Low;
    |         
    |     end
    |   
    | 
    | end
